simulink model "PD_EDDA"  (R2014b)
settings: Solver=ode23  StartTime=0.0  StopTime=100  RelTol=1e-10
values from neighbouring files (symbols this model uses):
  P = 1    [skrypt_EDDA.m]
settings Model: Creator=lab1.5  LastModifiedBy=Dawid Perdek

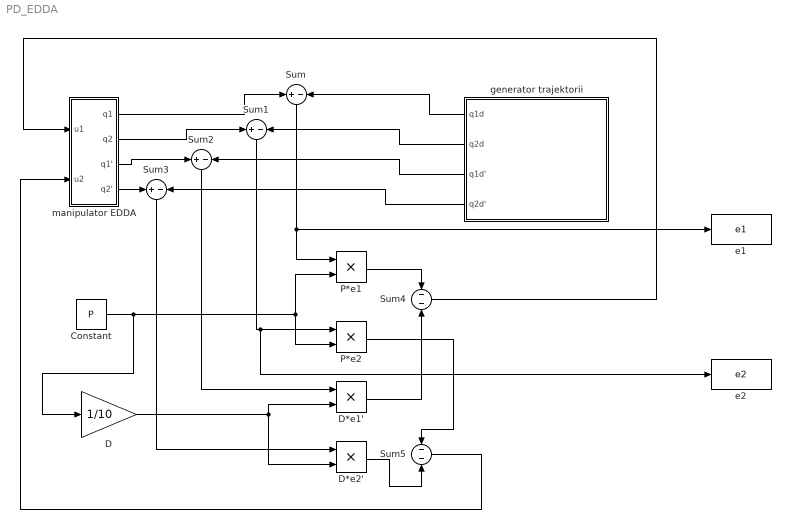
== system PD_EDDA ==
  Constant : Constant  Value=P
  D : Gain  Gain=1/10
  D*e1' : Product
  D*e2' : Product
  P*e1 : Product
  P*e2 : Product
  Sum{,1..3} (4 alike) : Sum  Inputs=+-
  Sum4 : Sum  Inputs=--
  Sum5 : Sum  Inputs=--
  e1 : ToWorkspace  VariableName=e1  SampleTime=-1
  e2 : ToWorkspace  VariableName=e2  SampleTime=-1
  generator trajektorii : Subsystem
  manipulator EDDA : Subsystem
  wires:
  manipulator EDDA/1(q1) -> Sum/1
  manipulator EDDA/2(q2) -> Sum1/1
  manipulator EDDA/3(q1') -> Sum2/1
  manipulator EDDA/4(q2') -> Sum3/1
  generator trajektorii/1(q1d) -> Sum/2
  generator trajektorii/2(q2d) -> Sum1/2
  generator trajektorii/3(q1d') -> Sum2/2
  generator trajektorii/4(q2d') -> Sum3/2
  Sum/1 -> P*e1/1, e1/1
  Sum2/1 -> D*e1'/1
  Sum3/1 -> D*e2'/1
  Constant/1 -> D/1, P*e2/2, P*e1/2
  D/1 -> D*e2'/2, D*e1'/2
  Sum4/1 -> manipulator EDDA/1(u1)
  Sum5/1 -> manipulator EDDA/2(u2)
  Sum1/1 -> e2/1, P*e2/1
  P*e1/1 -> Sum4/1
  D*e1'/1 -> Sum4/2
  P*e2/1 -> Sum5/1
  D*e2'/1 -> Sum5/2

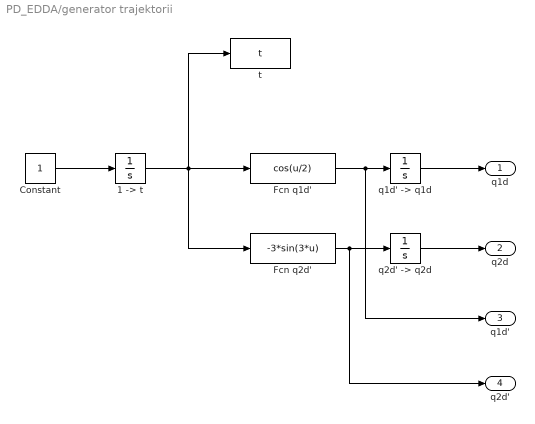
== system PD_EDDA/generator trajektorii ==
  "1 -> t" : Integrator
  Constant : Constant
  Fcn q1d' : Fcn  Expr=cos(u/2)
  Fcn q2d' : Fcn  Expr=-3*sin(3*u)
  "q1d' -> q1d" : Integrator
  "q2d' -> q2d" : Integrator  InitialCondition=1
  t : ToWorkspace  VariableName=t  SampleTime=-1
  q1d : Outport
  q2d : Outport  Port=2
  q1d' : Outport  Port=3
  q2d' : Outport  Port=4
  wires:
  Constant/1 -> "1 -> t"/1
  "1 -> t"/1 -> t/1, Fcn q2d'/1, Fcn q1d'/1
  Fcn q1d'/1 -> q1d'/1, "q1d' -> q1d"/1
  Fcn q2d'/1 -> q2d'/1, "q2d' -> q2d"/1
  "q1d' -> q1d"/1 -> q1d/1
  "q2d' -> q2d"/1 -> q2d/1

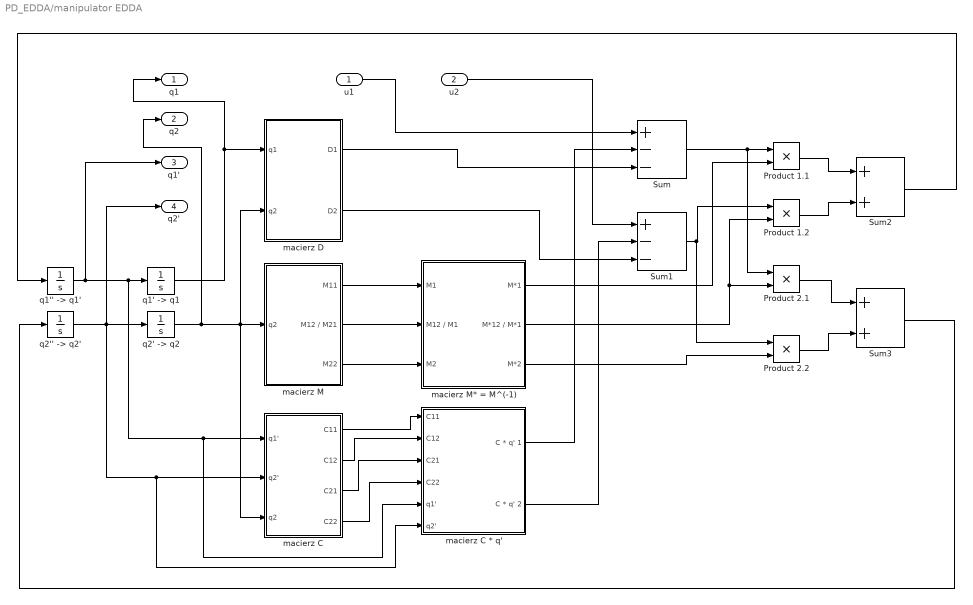
== system PD_EDDA/manipulator EDDA ==
  u1 : Inport
  u2 : Inport  Port=2
  Product 1.1 : Product
  Product 1.2 : Product
  Product 2.1 : Product
  Product 2.2 : Product
  Sum : Sum  Inputs=+--
  Sum1 : Sum  Inputs=+--
  Sum2 : Sum
  Sum3 : Sum
  macierz C : Subsystem
  macierz C * q' : Subsystem
  macierz D : Subsystem
  macierz M : Subsystem
  macierz M* = M^(-1) : Subsystem
  "q1' -> q1" : Integrator
  "q1'' -> q1'" : Integrator
  "q2' -> q2" : Integrator
  "q2'' -> q2'" : Integrator
  q1 : Outport
  q2 : Outport  Port=2
  q1' : Outport  Port=3
  q2' : Outport  Port=4
  wires:
  "q1'' -> q1'"/1 -> q1'/1, macierz C * q'/5(q1'), macierz C/1(q1'), "q1' -> q1"/1
  "q2'' -> q2'"/1 -> q2'/1, macierz C * q'/6(q2'), macierz C/2(q2'), "q2' -> q2"/1
  "q1' -> q1"/1 -> q1/1, macierz D/1(q1)
  "q2' -> q2"/1 -> q2/1, macierz C/3(q2), macierz D/2(q2), macierz M/1(q2)
  macierz C/1(C11) -> macierz C * q'/1(C11)
  macierz C/2(C12) -> macierz C * q'/2(C12)
  macierz C/3(C21) -> macierz C * q'/3(C21)
  macierz C/4(C22) -> macierz C * q'/4(C22)
  u1/1 -> Sum/1
  macierz C * q'/1(C * q' 1) -> Sum/2
  macierz D/1(D1) -> Sum/3
  u2/1 -> Sum1/1
  macierz C * q'/2(C * q' 2) -> Sum1/2
  macierz D/2(D2) -> Sum1/3
  Sum/1 -> Product 2.1/1, Product 1.1/1
  Sum1/1 -> Product 2.2/1, Product 1.2/1
  Product 1.1/1 -> Sum2/1
  Product 1.2/1 -> Sum2/2
  Product 2.1/1 -> Sum3/1
  Product 2.2/1 -> Sum3/2
  Sum2/1 -> "q1'' -> q1'"/1
  Sum3/1 -> "q2'' -> q2'"/1
  macierz M/1(M11) -> macierz M* = M^(-1)/1(M1)
  macierz M/2(M12 / M21) -> macierz M* = M^(-1)/2(M12 / M1)
  macierz M/3(M22) -> macierz M* = M^(-1)/3(M2)
  macierz M* = M^(-1)/1(M*1) -> Product 1.1/2
  macierz M* = M^(-1)/2(M*12 / M*1) -> Product 2.1/2, Product 1.2/2
  macierz M* = M^(-1)/3(M*2) -> Product 2.2/2

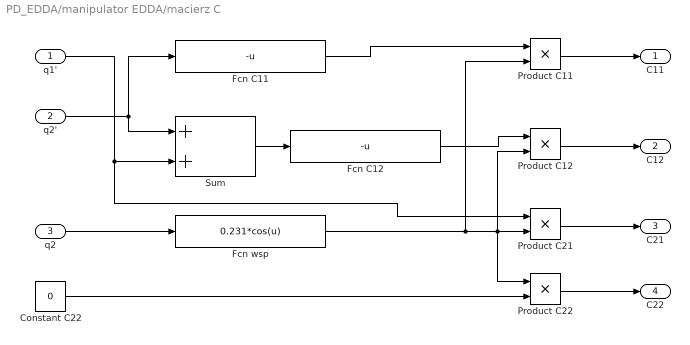
== system PD_EDDA/manipulator EDDA/macierz C ==
  q1' : Inport
  q2' : Inport  Port=2
  q2 : Inport  Port=3
  Constant C22 : Constant  Value=0
  Fcn C11 : Fcn  Expr=-u
  Fcn C12 : Fcn  Expr=-u
  Fcn wsp : Fcn  Expr=0.231*cos(u)
  Product C{11..12,21..22} (4 alike) : Product
  Sum : Sum
  C11 : Outport
  C12 : Outport  Port=2
  C21 : Outport  Port=3
  C22 : Outport  Port=4
  wires:
  q2/1 -> Fcn wsp/1
  Constant C22/1 -> Product C22/2
  Fcn wsp/1 -> Product C11/2, Product C12/2, Product C21/2, Product C22/1
  Product C22/1 -> C22/1
  q1'/1 -> Sum/2, Product C21/1
  Product C21/1 -> C21/1
  q2'/1 -> Sum/1, Fcn C11/1
  Fcn C11/1 -> Product C11/1
  Product C11/1 -> C11/1
  Sum/1 -> Fcn C12/1
  Product C12/1 -> C12/1
  Fcn C12/1 -> Product C12/1

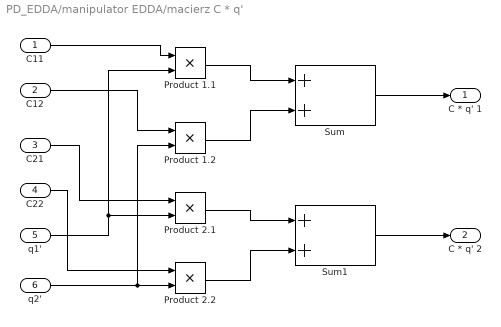
== system PD_EDDA/manipulator EDDA/macierz C * q' ==
  C11 : Inport
  C12 : Inport  Port=2
  C21 : Inport  Port=3
  C22 : Inport  Port=4
  q1' : Inport  Port=5
  q2' : Inport  Port=6
  Product 1.1 : Product
  Product 1.2 : Product
  Product 2.1 : Product
  Product 2.2 : Product
  Sum : Sum
  Sum1 : Sum
  C * q' 1 : Outport
  C * q' 2 : Outport  Port=2
  wires:
  C11/1 -> Product 1.1/1
  q1'/1 -> Product 2.1/2, Product 1.1/2
  C12/1 -> Product 1.2/1
  q2'/1 -> Product 2.2/2, Product 1.2/2
  Product 1.1/1 -> Sum/1
  Product 1.2/1 -> Sum/2
  Sum/1 -> C * q' 1/1
  C21/1 -> Product 2.1/1
  C22/1 -> Product 2.2/1
  Product 2.1/1 -> Sum1/1
  Product 2.2/1 -> Sum1/2
  Sum1/1 -> C * q' 2/1

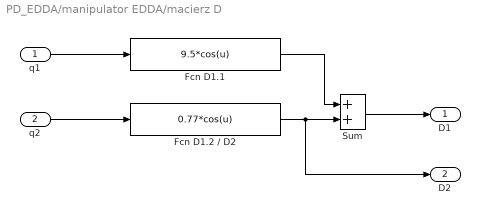
== system PD_EDDA/manipulator EDDA/macierz D ==
  q1 : Inport
  q2 : Inport  Port=2
  Fcn D1.1 : Fcn  Expr=9.5*cos(u)
  Fcn D1.2 / D2 : Fcn  Expr=0.77*cos(u)
  Sum : Sum
  D1 : Outport
  D2 : Outport  Port=2
  wires:
  q2/1 -> Fcn D1.2 / D2/1
  q1/1 -> Fcn D1.1/1
  Fcn D1.2 / D2/1 -> D2/1, Sum/2
  Fcn D1.1/1 -> Sum/1
  Sum/1 -> D1/1

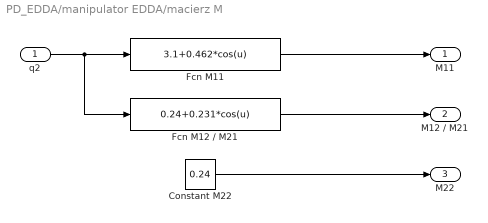
== system PD_EDDA/manipulator EDDA/macierz M ==
  q2 : Inport
  Constant M22 : Constant  Value=0.24
  Fcn M11 : Fcn  Expr=3.1+0.462*cos(u)
  Fcn M12 / M21 : Fcn  Expr=0.24+0.231*cos(u)
  M11 : Outport
  M12 / M21 : Outport  Port=2
  M22 : Outport  Port=3
  wires:
  Fcn M12 / M21/1 -> M12 / M21/1
  Fcn M11/1 -> M11/1
  q2/1 -> Fcn M12 / M21/1, Fcn M11/1
  Constant M22/1 -> M22/1

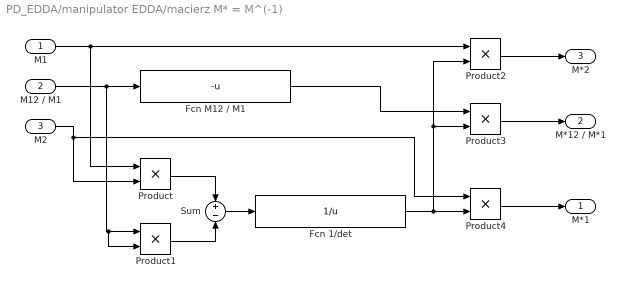
== system PD_EDDA/manipulator EDDA/macierz M* = M^(-1) ==
  M1 : Inport
  M12 / M1 : Inport  Port=2
  M2 : Inport  Port=3
  Fcn 1/det : Fcn  Expr=1/u
  Fcn M12 / M1 : Fcn  Expr=-u
  Product{,1..4} (5 alike) : Product
  Sum : Sum  Inputs=+-
  M*1 : Outport
  M*12 / M*1 : Outport  Port=2
  M*2 : Outport  Port=3
  wires:
  M2/1 -> Product4/1, Product/2
  M1/1 -> Product2/1, Product/1
  M12 / M1/1 -> Product1/2, Product1/1, Fcn M12 / M1/1
  Product/1 -> Sum/1
  Product1/1 -> Sum/2
  Sum/1 -> Fcn 1/det/1
  Fcn 1/det/1 -> Product4/2, Product2/2, Product3/2
  Fcn M12 / M1/1 -> Product3/1
  Product2/1 -> M*2/1
  Product3/1 -> M*12 / M*1/1
  Product4/1 -> M*1/1
